simulink model "exemplo_bloco_modelo"  (R2024b)
settings: Solver=ode45  StartTime=0.0  StopTime=200  FixedStep=0.0005  RelTol=1e-6
undefined symbols (not defined in the file): MODEL
settings Model: Creator=Mauricio  LastModifiedBy=johne
settings SolverCC: AlgebraicLoopSolver=TrustRegion
settings DataIOCC: LimitDataPoints=on  SaveFormat=Array  ReturnWorkspaceOutputs=off
settings OptimizationCC: InitFltsAndDblsToZero=on  LifeSpan=inf
settings DebuggingCC: SaveWithParameterizedLinksMsg=none  SignalResolutionControl=TryResolveAllWithWarning  SolverPrmCheckMsg=warning  MultiTaskDSMMsg=warning  MultiTaskCondExecSysMsg=none  FcnCallInpInsideContextMsg=warning  UnconnectedInputMsg=warning  UnconnectedOutputMsg=warning  UnconnectedLineMsg=warning  SFUnexpectedBacktrackingDiag=warning  SFNoUnconditionalDefaultTransitionDiag=warning  SFExecutionAtInitializationDiag=none  ArithmeticOperatorsInVariantConditions=warning
settings HardwareCC: ProdBitPerPointer=32  ProdBitPerSizeT=32  ProdBitPerPtrDiffT=32  ProdLargestAtomicFloat=None  ProdIntDivRoundTo=Undefined  ProdEndianess=Unspecified  ProdWordSize=32  ProdHWDeviceType=32-bit Generic
settings ModelReferenceCC: EnableRefExpFcnMdlSchedulingChecks=on  PropagateSignalLabelsOutOfModel=off
settings SFSimCC: SimUseLocalCustomCode=off  CustomCodeUndefinedFunction=UseInterfaceOnly
settings RTWCC: RTWUseLocalCustomCode=off  GPUComputeCapability=3.5
settings CodeAppCC: StateflowObjectComments=on
settings GRTTargetCC: TargetFcnLib=ansi_tfl_tmw.mat  TargetLangStandard=C89/C90 (ANSI)  CombineOutputUpdateFcns=off  GRTInterface=on
settings ConfigComp: CovMetricSettings=dw  CovSaveCumulativeToWorkspaceVar=on  CovSaveSingleToWorkspaceVar=on  CovExternalEMLEnable=off  CovSFcnEnable=off

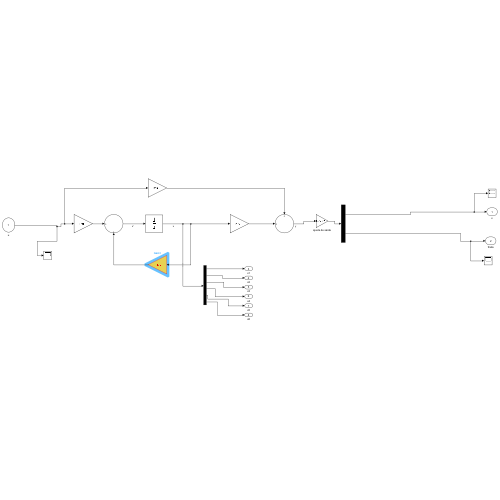
[thumbnail: Simulink's stored preview of the top-level diagram]
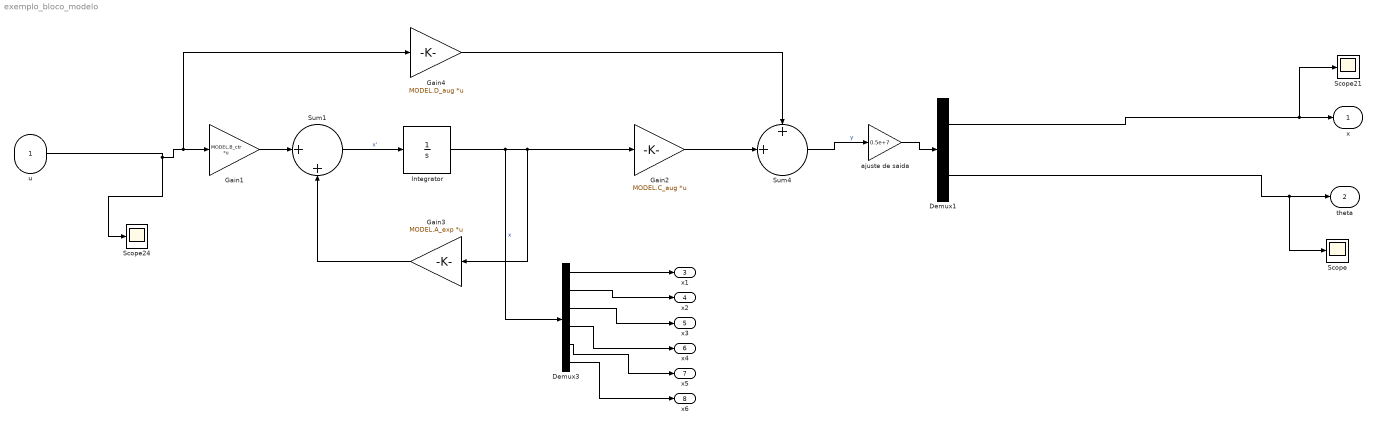
== system exemplo_bloco_modelo ==
  u : Inport
  Demux1 : Demux  Outputs=2
  Demux3 : Demux  Outputs=6
  Gain1 : Gain  Gain=MODEL.B_ctr  Multiplication=Matrix(K*u)
  Gain2 : Gain  Gain=MODEL.C_aug  Multiplication=Matrix(K*u)
  Gain3 : Gain  Gain=MODEL.A_exp  Multiplication=Matrix(K*u)
  Gain4 : Gain  Gain=MODEL.D_aug  Multiplication=Matrix(K*u)
  Integrator : Integrator
  Scope : Scope
  Scope21 : Scope
  Scope24 : Scope
  Sum1 : Sum  Inputs=|++
  Sum4 : Sum  Inputs=++|
  ajuste de saida : Gain  Gain=0.5e+7
  x : Outport  VectorParamsAs1DForOutWhenUnconnected=off
  theta : Outport  Port=2  VectorParamsAs1DForOutWhenUnconnected=off
  x1 : Outport  Port=3
  x2 : Outport  Port=4
  x3 : Outport  Port=5
  x4 : Outport  Port=6
  x5 : Outport  Port=7
  x6 : Outport  Port=8
  wires:
  Gain4/1 -> Sum4/1
  Demux3/1 -> x1/1
  u/1 -> Scope24/1, Gain4/1, Gain1/1
  Demux3/6 -> x6/1
  Demux3/5 -> x5/1
  Gain2/1 -> Sum4/2
  Gain1/1 -> Sum1/1
  Demux3/2 -> x2/1
  Integrator/1 -> Demux3/1, Gain3/1, Gain2/1  "x"
  Demux3/4 -> x4/1
  Demux1/1 -> Scope21/1, x/1
  Demux1/2 -> Scope/1, theta/1
  Demux3/3 -> x3/1
  Gain3/1 -> Sum1/2
  Sum4/1 -> ajuste de saida/1  "y"
  Sum1/1 -> Integrator/1  "x'"
  ajuste de saida/1 -> Demux1/1
